simulink model "SuspensionStateSpaceModel"  (R2018a)
settings: Solver=VariableStepAuto  StartTime=0.0  StopTime=5  MaxStep=0.025  RelTol=1e-3  AbsTol=1e-3
values from neighbouring files (symbols this model uses):
  A = [0 1 0 0 ... (first row only)    [Algoritmo_gen.m]
  B = [0; [(c2/m2)*(c1/m1)]; -c1/m1; -k1/m1]    [Algoritmo_gen.m]    (also in Parametros_Susp_Ativa_GALQR.m = [0; [(bs11/m22)*(bp11/m11)]; -bp11/m11; -kp11/m11])
  K2 = lqr(A,B,Q1,R1)    [Algoritmo_gen.m]    (also in custo_gen.m)
undefined symbols (not defined in the file or in its folder): K, K1
settings Model: Creator=jeffersongomes  LastModifiedBy=jeffersongomes
settings SimscapeCC: SimscapeLogType=all  SimscapeLogOpenViewer=on

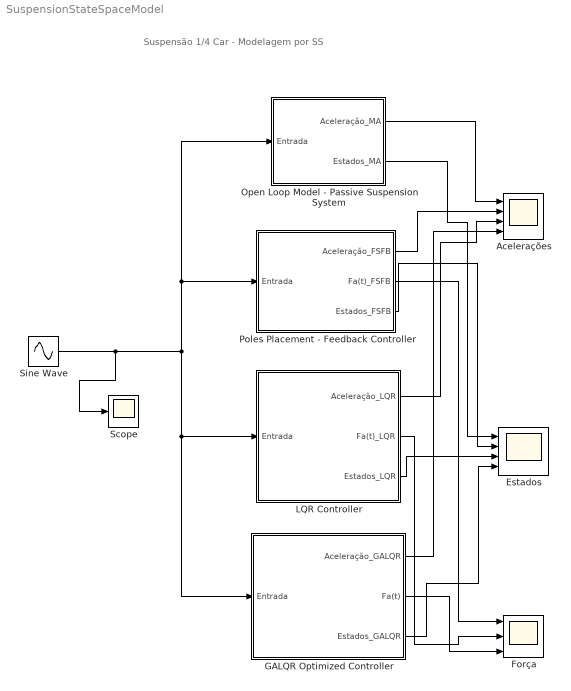
== system SuspensionStateSpaceModel ==
  note: Suspensão 1/4 Car - Modelagem por SS
  Acelerações : Scope  NumInputPorts=4
  Estados : Scope  NumInputPorts=4
  Força : Scope  NumInputPorts=3
  "GALQR Optimized Controller " : Subsystem
  "LQR Controller " : Subsystem
  Open Loop Model - Passive Suspension System : Subsystem
  Poles Placement - Feedback Controller : Subsystem
  Scope : Scope
  Sine Wave : Sin  Amplitude=0.30  Frequency=4.9  SampleTime=0
  wires:
  Poles Placement - Feedback Controller/1(Aceleração_FSFB) -> Acelerações/2
  Poles Placement - Feedback Controller/2(Fa(t)_FSFB) -> Força/1
  Poles Placement - Feedback Controller/3(Estados_FSFB) -> Estados/2
  "LQR Controller "/1(Aceleração_LQR) -> Acelerações/3
  "LQR Controller "/2(Fa(t)_LQR) -> Força/2
  "LQR Controller "/3(Estados_LQR) -> Estados/3
  "GALQR Optimized Controller "/1(Aceleração_GALQR) -> Acelerações/4
  "GALQR Optimized Controller "/2(Fa(t)) -> Força/3
  "GALQR Optimized Controller "/3(Estados_GALQR) -> Estados/4
  Open Loop Model - Passive Suspension System/1(Aceleração_MA) -> Acelerações/1
  Open Loop Model - Passive Suspension System/2(Estados_MA) -> Estados/1
  Sine Wave/1 -> Scope/1, "GALQR Optimized Controller "/1(Entrada), "LQR Controller "/1(Entrada), Poles Placement - Feedback Controller/1(Entrada), Open Loop Model - Passive Suspension System/1(Entrada)

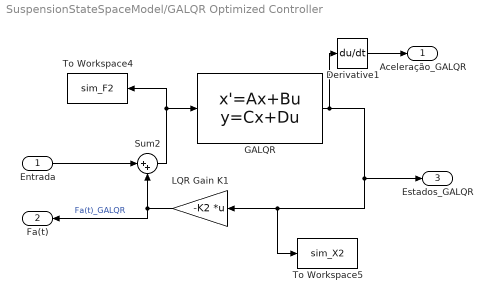
== system SuspensionStateSpaceModel/GALQR Optimized Controller  ==
  Entrada : Inport
  Derivative1 : Derivative
  GALQR : StateSpace  A=A  B=B  C=eye(4)  D=zeros(4,1)  InitialCondition=0
  LQR Gain K1 : Gain  Gain=-K2  Multiplication=Matrix(K*u)
  Sum2 : Sum  Inputs=|++
  To Workspace4 : ToWorkspace  VariableName=sim_F2  SaveFormat=Structure With Time  SampleTime=-1
  To Workspace5 : ToWorkspace  VariableName=sim_X2  SaveFormat=Structure With Time  SampleTime=-1
  Aceleração_GALQR : Outport
  Fa(t) : Outport  Port=2
  Estados_GALQR : Outport  Port=3
  wires:
  GALQR/1 -> Estados_GALQR/1, LQR Gain K1/1, To Workspace5/1, Derivative1/1
  Sum2/1 -> GALQR/1, To Workspace4/1
  Entrada/1 -> Sum2/1
  Derivative1/1 -> Aceleração_GALQR/1
  LQR Gain K1/1 -> Fa(t)/1, Sum2/2  "Fa(t)_GALQR"

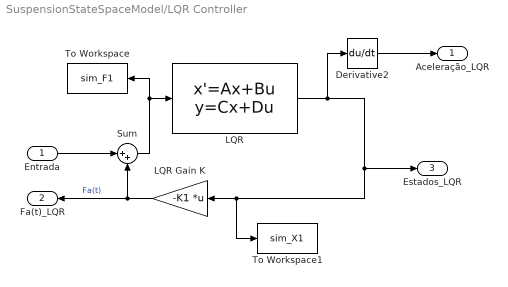
== system SuspensionStateSpaceModel/LQR Controller  ==
  Entrada : Inport
  Derivative2 : Derivative
  LQR : StateSpace  A=A  B=B  C=eye(4)  D=zeros(4,1)  InitialCondition=0
  LQR Gain K : Gain  Gain=-K1  Multiplication=Matrix(K*u)
  Sum : Sum  Inputs=|++
  To Workspace : ToWorkspace  VariableName=sim_F1  SaveFormat=Structure With Time  SampleTime=-1
  To Workspace1 : ToWorkspace  VariableName=sim_X1  SaveFormat=Structure With Time  SampleTime=-1
  Aceleração_LQR : Outport
  Fa(t)_LQR : Outport  Port=2
  Estados_LQR : Outport  Port=3
  wires:
  Sum/1 -> LQR/1, To Workspace/1
  LQR Gain K/1 -> Fa(t)_LQR/1, Sum/2  "Fa(t)"
  LQR/1 -> Derivative2/1, Estados_LQR/1, To Workspace1/1, LQR Gain K/1
  Derivative2/1 -> Aceleração_LQR/1
  Entrada/1 -> Sum/1

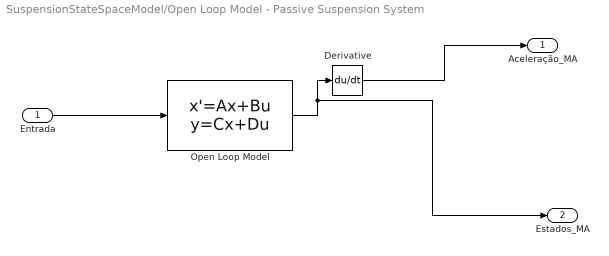
== system SuspensionStateSpaceModel/Open Loop Model - Passive Suspension System ==
  Entrada : Inport
  Derivative : Derivative
  Open Loop Model : StateSpace  A=A  B=B  C=eye(4)  D=zeros(4,1)  InitialCondition=0
  Aceleração_MA : Outport
  Estados_MA : Outport  Port=2
  wires:
  Open Loop Model/1 -> Estados_MA/1, Derivative/1
  Derivative/1 -> Aceleração_MA/1
  Entrada/1 -> Open Loop Model/1

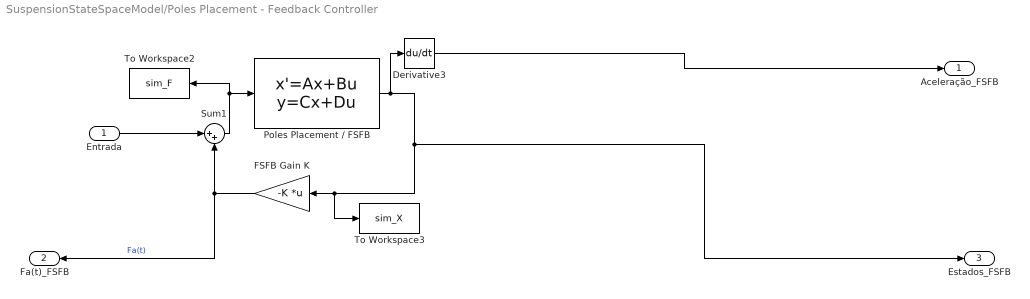
== system SuspensionStateSpaceModel/Poles Placement - Feedback Controller ==
  Entrada : Inport
  Derivative3 : Derivative
  FSFB Gain K : Gain  Gain=-K  Multiplication=Matrix(K*u)
  Poles Placement / FSFB : StateSpace  A=A  B=B  C=eye(4)  D=zeros(4,1)  InitialCondition=0
  Sum1 : Sum  Inputs=|++
  To Workspace2 : ToWorkspace  VariableName=sim_F  SaveFormat=Structure With Time  SampleTime=-1
  To Workspace3 : ToWorkspace  VariableName=sim_X  SaveFormat=Structure With Time  SampleTime=-1
  Aceleração_FSFB : Outport
  Fa(t)_FSFB : Outport  Port=2
  Estados_FSFB : Outport  Port=3
  wires:
  Entrada/1 -> Sum1/1
  FSFB Gain K/1 -> Fa(t)_FSFB/1, Sum1/2  "Fa(t)"
  Derivative3/1 -> Aceleração_FSFB/1
  Poles Placement / FSFB/1 -> Estados_FSFB/1, FSFB Gain K/1, To Workspace3/1, Derivative3/1
  Sum1/1 -> Poles Placement / FSFB/1, To Workspace2/1
